simulink model "final_robot_model"  (R2023b)
settings: Solver=VariableStepAuto  StartTime=0.0  StopTime=10.0  RelTol=1e-3
values from neighbouring files (symbols this model uses):
  acceleration_limit = 3    [parameters.m]
  D = 0.93e-6    (= 9.3e-07)    [parameters.m]
  dist0 = 0    [parameters.m]
  gear = 9.6    [parameters.m]
  heading_ref = 0.9    [parameters.m]    (also in set_and_go.m = deg2rad(heading_ref_deg))
  J = 1.01e-6    (= 1.01e-06)    [parameters.m]
  Kb = 0.0074    [parameters.m]
  Kt = Kb    (= 0.0074)    [parameters.m]
  L = 4.1e-3    (= 0.0041)    [parameters.m]
  M = 0.95    [parameters.m]
  path = path .* 0.1    [parameters.m]
  R = 4.1    [parameters.m]
  theta0 = 0    [parameters.m]
  transport_delay = 0.01    [parameters.m]
  Ts = 0.004    [parameters.m]
  turn_acc_limit = 5    [parameters.m]
  vel_ref = 0.5    [parameters.m]
  wheel_distance = 0.147    [parameters.m]
  wrad = 0.03    [parameters.m]
  wzi = (0.065)^2 * M    (= 0.00401375)    [parameters.m]
  x0 = 0    [parameters.m]    (also in plot_trajectory.m = evalin("base", "x0"))
  y0 = 0    [parameters.m]    (also in plot_trajectory.m = evalin("base", "y0"))
undefined symbols (not defined in the file or in its folder): alpha, alpha_heading, Ki, Ki_heading, Ki_turnrate, Kp, Kp_heading, Kp_turnrate, taud, taud_heading
settings Model: Creator=Gianluca  LastModifiedBy=simone

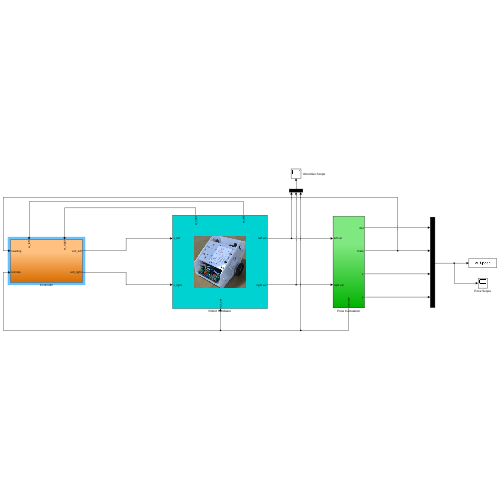
[thumbnail: Simulink's stored preview of the top-level diagram]
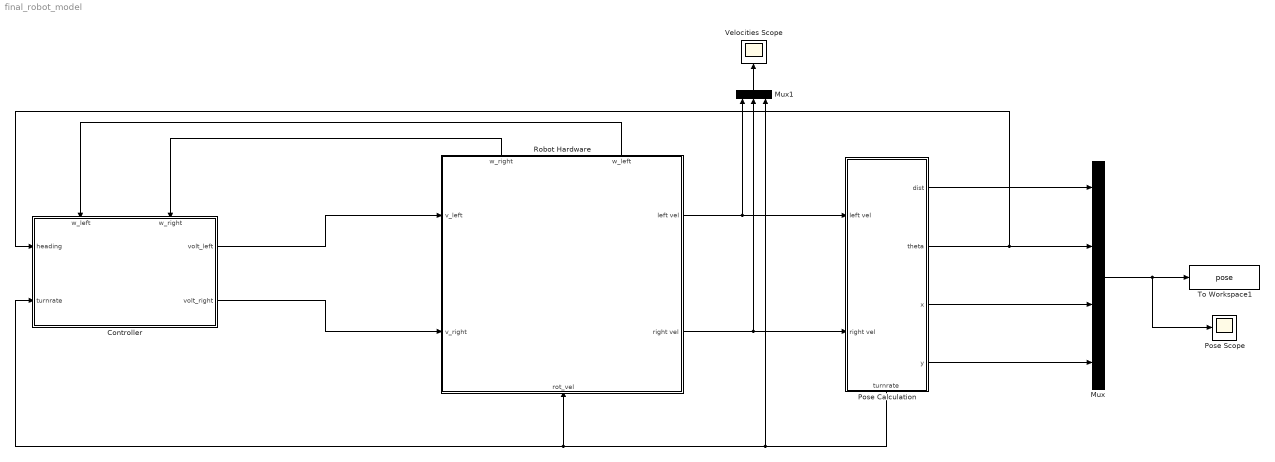
== system final_robot_model ==
  Controller : Subsystem
      settings: PortSchema="{\"entries\":[{\"content\":{\"sides\":[{\"content\":{\"connectorIds\":[\"In1\",\"In2\"]},\"type\":\"ConnectorPlacement.EquallySpacedRectSide\",\"uuid\":\"3d11a138-6336-4e96-9bd3-dfa953b9eab0\"},{\"content\":{\"connectorIds\":[\"Out1\",\"Out2\"],\"side\":\"RIGHT\"},\"type\":\"ConnectorPlacement.EquallySpacedRectSide\",\"uuid\":\"de9a8172-5842-4792-a376-2910158aed35\"},{\"content\":{\"connectorIds\":[\"In3\",\"In4\"],\"side\":\"TOP\"},\"type\":\"ConnectorPlacement.EquallySpacedRectSide\",\"uuid\":\"81659c89-c220-4746-8992-e8ba86bf75e6\"},{\"content\":{\"side\":\"BOTTOM\"},\"type\":\"ConnectorPlacement.EquallySpacedRectSide\",\"uuid\":\"e4167768-df9a-443c-9e0f-b27adaafe9f8\"}]},\"type\":\"ConnectorPlacement.EquallySpacedConnector\",\"uuid\":\"b42d2ec0-7f18-44e6-b925-f5795e7bb3dd\"}],\"packageUris\":[\"http://schema.mathworks.com/mf0/Connector/R2020b\"],\"version\":\"1.0\"}"
  Mux : Mux
  Mux1 : Mux  Inputs=3
  Pose Calculation : Subsystem
      settings: PortSchema="{\"entries\":[{\"content\":{\"sides\":[{\"content\":{\"connectorIds\":[\"In1\",\"In2\"]},\"type\":\"ConnectorPlacement.EquallySpacedRectSide\",\"uuid\":\"46289eb4-3bbb-404a-99f0-e253fad6e87f\"},{\"content\":{\"connectorIds\":[\"Out1\",\"Out2\",\"Out3\",\"Out4\"],\"side\":\"RIGHT\"},\"type\":\"ConnectorPlacement.EquallySpacedRectSide\",\"uuid\":\"ccfc4e76-4e0e-4fcd-8da4-ce03e19c701c\"},{\"content\":{\"side\":\"TOP\"},\"type\":\"ConnectorPlacement.EquallySpacedRectSide\",\"uuid\":\"be5e5684-5a07-4d94-a4cd-7af4c2fd824b\"},{\"content\":{\"connectorIds\":[\"Out5\"],\"side\":\"BOTTOM\"},\"type\":\"ConnectorPlacement.EquallySpacedRectSide\",\"uuid\":\"f3a7bad1-4db8-4eb0-a537-6e6993dfbfe6\"}]},\"type\":\"ConnectorPlacement.EquallySpacedConnector\",\"uuid\":\"6a4a9bee-79c3-4932-b89c-a6fb8d0f2d92\"}],\"packageUris\":[\"http://schema.mathworks.com/mf0/Connector/R2020b\"],\"version\":\"1.0\"}"
  Pose Scope : Scope
  Robot Hardware : Subsystem
      settings: PortSchema="{\"entries\":[{\"content\":{\"sides\":[{\"content\":{\"connectorIds\":[\"In1\",\"In2\"]},\"type\":\"ConnectorPlacement.EquallySpacedRectSide\",\"uuid\":\"419fea77-f9ca-4e06-bea6-681a18650ab8\"},{\"content\":{\"connectorIds\":[\"Out1\",\"Out2\"],\"side\":\"RIGHT\"},\"type\":\"ConnectorPlacement.EquallySpacedRectSide\",\"uuid\":\"1629cad4-6101-470f-acc1-fad0cb327def\"},{\"content\":{\"connectorIds\":[\"Out3\",\"Out4\"],\"side\":\"TOP\"},\"type\":\"ConnectorPlacement.EquallySpacedRectSide\",\"uuid\":\"70c90e71-c188-4b9c-b220-781da08827f9\"},{\"content\":{\"connectorIds\":[\"In3\"],\"side\":\"BOTTOM\"},\"type\":\"ConnectorPlacement.EquallySpacedRectSide\",\"uuid\":\"6ff6b814-ff30-4b88-82ef-7ebf956f2560\"}]},\"type\":\"ConnectorPlacement.EquallySpacedConnector\",\"uuid\":\"ad56978f-143c-418e-863d-6c6f1f6f5d0c\"}],\"packageUris\":[\"http://schema.mathworks.com/mf0/Connector/R2020b\"],\"version\":\"1.0\"}"
      mask Display: image('regbot.png');
  To Workspace1 : ToWorkspace  VariableName=pose  SaveFormat=Timeseries  SampleTime=-1
  Velocities Scope : Scope
  wires:
  Pose Calculation/5(turnrate) -> Mux1/3, Robot Hardware/3(rot_vel), Controller/2(turnrate)
  Mux/1 -> To Workspace1/1, Pose Scope/1
  Pose Calculation/2(theta) -> Mux/2, Controller/1(heading)
  Pose Calculation/1(dist) -> Mux/1
  Mux1/1 -> Velocities Scope/1
  Pose Calculation/3(x) -> Mux/3
  Pose Calculation/4(y) -> Mux/4
  Robot Hardware/4(w_left) -> Controller/3(w_left)
  Robot Hardware/3(w_right) -> Controller/4(w_right)
  Controller/1(volt_left) -> Robot Hardware/1(v_left)
  Controller/2(volt_right) -> Robot Hardware/2(v_right)
  Robot Hardware/1(left vel) -> Pose Calculation/1(left vel), Mux1/1
  Robot Hardware/2(right vel) -> Pose Calculation/2(right vel), Mux1/2

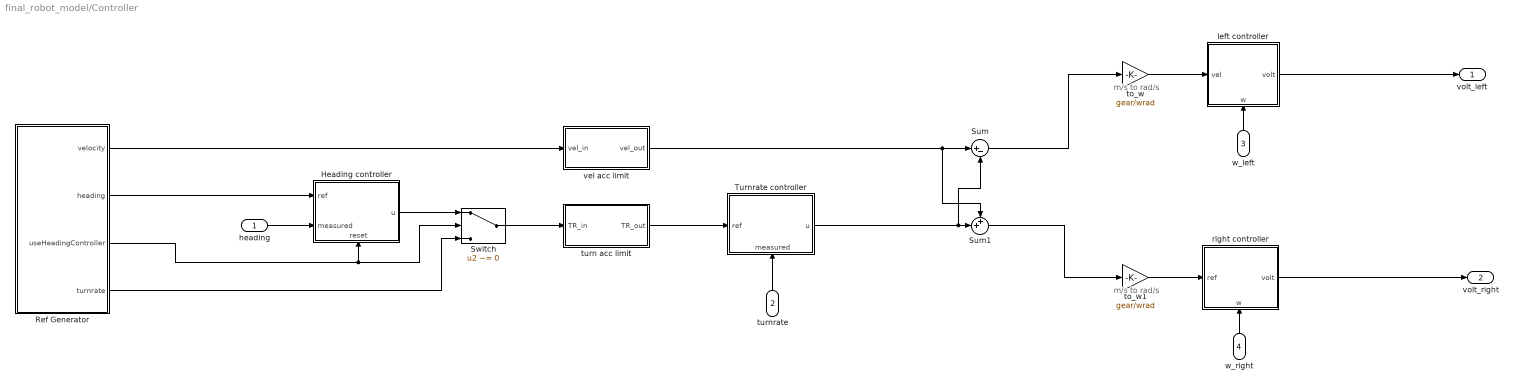
== system final_robot_model/Controller ==
  note: m/s to rad/s
  note: m/s to rad/s
  heading : Inport
  turnrate : Inport  Port=2
  w_left : Inport  Port=3
  w_right : Inport  Port=4
  Heading controller : Subsystem
      settings: PortSchema="{\"entries\":[{\"content\":{\"sides\":[{\"content\":{\"connectorIds\":[\"In1\",\"In2\"]},\"type\":\"ConnectorPlacement.EquallySpacedRectSide\",\"uuid\":\"3bde791d-a2ac-4d13-a51a-30874ee8f75a\"},{\"content\":{\"connectorIds\":[\"Out1\"],\"side\":\"RIGHT\"},\"type\":\"ConnectorPlacement.EquallySpacedRectSide\",\"uuid\":\"88ae4683-d3e7-483e-be55-3d26372f5fe2\"},{\"content\":{\"side\":\"TOP\"},\"type\":\"ConnectorPlacement.EquallySpacedRectSide\",\"uuid\":\"26752a72-f697-4de9-9dcd-1ca4cee0df39\"},{\"content\":{\"connectorIds\":[\"In3\"],\"side\":\"BOTTOM\"},\"type\":\"ConnectorPlacement.EquallySpacedRectSide\",\"uuid\":\"98a7b674-7c45-4a73-92a3-8750bdde1f36\"}]},\"type\":\"ConnectorPlacement.EquallySpacedConnector\",\"uuid\":\"d259c3e3-c5d7-42b6-881b-3a633aa969c6\"}],\"packageUris\":[\"http://schema.mathworks.com/mf0/Connector/R2020b\"],\"version\":\"1.0\"}"
  Ref Generator : Subsystem
  Sum : Sum  Inputs=|+-
  Sum1 : Sum  Inputs=++|
  Switch : Switch  Criteria=u2 ~= 0  Threshold=-999999  SaturateOnIntegerOverflow=off  InputSameDT=off
  Turnrate controller : Subsystem
      settings: PortSchema="{\"entries\":[{\"content\":{\"sides\":[{\"content\":{\"connectorIds\":[\"In1\"]},\"type\":\"ConnectorPlacement.EquallySpacedRectSide\",\"uuid\":\"3bde791d-a2ac-4d13-a51a-30874ee8f75a\"},{\"content\":{\"connectorIds\":[\"Out1\"],\"side\":\"RIGHT\"},\"type\":\"ConnectorPlacement.EquallySpacedRectSide\",\"uuid\":\"88ae4683-d3e7-483e-be55-3d26372f5fe2\"},{\"content\":{\"side\":\"TOP\"},\"type\":\"ConnectorPlacement.EquallySpacedRectSide\",\"uuid\":\"26752a72-f697-4de9-9dcd-1ca4cee0df39\"},{\"content\":{\"connectorIds\":[\"In2\"],\"side\":\"BOTTOM\"},\"type\":\"ConnectorPlacement.EquallySpacedRectSide\",\"uuid\":\"98a7b674-7c45-4a73-92a3-8750bdde1f36\"}]},\"type\":\"ConnectorPlacement.EquallySpacedConnector\",\"uuid\":\"d259c3e3-c5d7-42b6-881b-3a633aa969c6\"}],\"packageUris\":[\"http://schema.mathworks.com/mf0/Connector/R2020b\"],\"version\":\"1.0\"}"
  left controller : Subsystem
      settings: PortSchema="{\"entries\":[{\"content\":{\"sides\":[{\"content\":{\"connectorIds\":[\"In1\"]},\"type\":\"ConnectorPlacement.EquallySpacedRectSide\",\"uuid\":\"3bde791d-a2ac-4d13-a51a-30874ee8f75a\"},{\"content\":{\"connectorIds\":[\"Out1\"],\"side\":\"RIGHT\"},\"type\":\"ConnectorPlacement.EquallySpacedRectSide\",\"uuid\":\"88ae4683-d3e7-483e-be55-3d26372f5fe2\"},{\"content\":{\"side\":\"TOP\"},\"type\":\"ConnectorPlacement.EquallySpacedRectSide\",\"uuid\":\"26752a72-f697-4de9-9dcd-1ca4cee0df39\"},{\"content\":{\"connectorIds\":[\"In2\"],\"side\":\"BOTTOM\"},\"type\":\"ConnectorPlacement.EquallySpacedRectSide\",\"uuid\":\"8837b86a-35cd-4679-9975-e69b760c287c\"}]},\"type\":\"ConnectorPlacement.EquallySpacedConnector\",\"uuid\":\"d259c3e3-c5d7-42b6-881b-3a633aa969c6\"}],\"packageUris\":[\"http://schema.mathworks.com/mf0/Connector/R2020b\"],\"version\":\"1.0\"}"
  right controller : Subsystem
      settings: PortSchema="{\"entries\":[{\"content\":{\"sides\":[{\"content\":{\"connectorIds\":[\"In1\"]},\"type\":\"ConnectorPlacement.EquallySpacedRectSide\",\"uuid\":\"3bde791d-a2ac-4d13-a51a-30874ee8f75a\"},{\"content\":{\"connectorIds\":[\"Out1\"],\"side\":\"RIGHT\"},\"type\":\"ConnectorPlacement.EquallySpacedRectSide\",\"uuid\":\"88ae4683-d3e7-483e-be55-3d26372f5fe2\"},{\"content\":{\"side\":\"TOP\"},\"type\":\"ConnectorPlacement.EquallySpacedRectSide\",\"uuid\":\"26752a72-f697-4de9-9dcd-1ca4cee0df39\"},{\"content\":{\"connectorIds\":[\"In2\"],\"side\":\"BOTTOM\"},\"type\":\"ConnectorPlacement.EquallySpacedRectSide\",\"uuid\":\"1adabdfb-f360-4bb8-8b57-8160c74899b3\"}]},\"type\":\"ConnectorPlacement.EquallySpacedConnector\",\"uuid\":\"d259c3e3-c5d7-42b6-881b-3a633aa969c6\"}],\"packageUris\":[\"http://schema.mathworks.com/mf0/Connector/R2020b\"],\"version\":\"1.0\"}"
  to_w : Gain  Gain=gear/wrad
  to_w1 : Gain  Gain=gear/wrad
  turn acc limit : Subsystem
  vel acc limit : Subsystem
  volt_left : Outport
  volt_right : Outport  Port=2
  wires:
  turn acc limit/1(TR_out) -> Turnrate controller/1(ref)
  left controller/1(volt) -> volt_left/1
  Turnrate controller/1(u) -> Sum/2, Sum1/2
  heading/1 -> Heading controller/2(measured)
  to_w/1 -> left controller/1(vel)
  Sum/1 -> to_w/1
  w_right/1 -> right controller/2(w)
  turnrate/1 -> Turnrate controller/2(measured)
  to_w1/1 -> right controller/1(ref)
  right controller/1(volt) -> volt_right/1
  Sum1/1 -> to_w1/1
  w_left/1 -> left controller/2(w)
  vel acc limit/1(vel_out) -> Sum1/1, Sum/1
  Ref Generator/2(heading) -> Heading controller/1(ref)
  Heading controller/1(u) -> Switch/1
  Switch/1 -> turn acc limit/1(TR_in)
  Ref Generator/4(turnrate) -> Switch/3
  Ref Generator/3(useHeadingController) -> Switch/2, Heading controller/3(reset)
  Ref Generator/1(velocity) -> vel acc limit/1(vel_in)

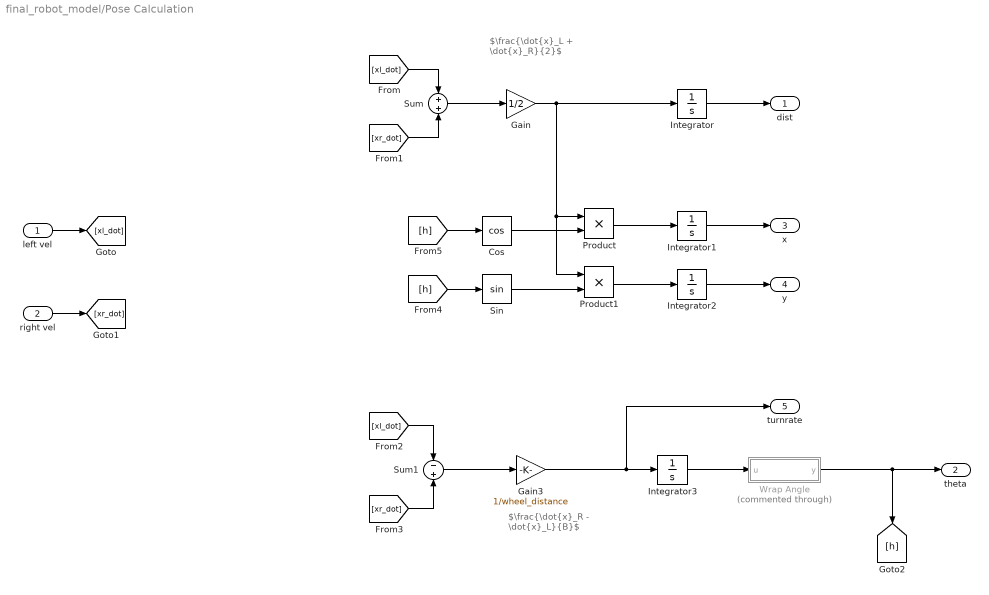
== system final_robot_model/Pose Calculation ==
  note: $\frac{\dot{x}_L + \dot{x}_R}{2}$
  note: $\frac{\dot{x}_R - \dot{x}_L}{B}$
  left vel : Inport
  right vel : Inport  Port=2
  Cos : Trigonometry  Operator=cos
  Gain : Gain  Gain=1/2
  Gain3 : Gain  Gain=1/wheel_distance
  Integrator : Integrator  InitialCondition=dist0
  Integrator1 : Integrator  InitialCondition=x0
  Integrator2 : Integrator  InitialCondition=y0
  Integrator3 : Integrator  InitialCondition=theta0
  Product : Product
  Product1 : Product
  Sin : Trigonometry
  Sum : Sum  Inputs=+|+
  Sum1 : Sum  Inputs=-|+
  Wrap Angle : MATLAB Function  Commented=through  TreatAsAtomicUnit=on
  dist : Outport
  theta : Outport  Port=2
  x : Outport  Port=3
  y : Outport  Port=4
  turnrate : Outport  Port=5
  wires:
  Sum/1 -> Gain/1
  Gain/1 -> Integrator/1, Product/1, Product1/1
  Integrator/1 -> dist/1
  left vel/1 -> [xl_dot]
  right vel/1 -> [xr_dot]
  [xl_dot] -> Sum/1
  [xr_dot] -> Sum/2
  [xl_dot] -> Sum1/1
  [xr_dot] -> Sum1/2
  Gain3/1 -> turnrate/1, Integrator3/1
  Sum1/1 -> Gain3/1
  [h] -> Sin/1
  Integrator2/1 -> y/1
  Integrator1/1 -> x/1
  [h] -> Cos/1
  Sin/1 -> Product1/2
  Cos/1 -> Product/2
  Product1/1 -> Integrator2/1
  Product/1 -> Integrator1/1
  Integrator3/1 -> Wrap Angle/1(u)
  Wrap Angle/1(y) -> [h], theta/1

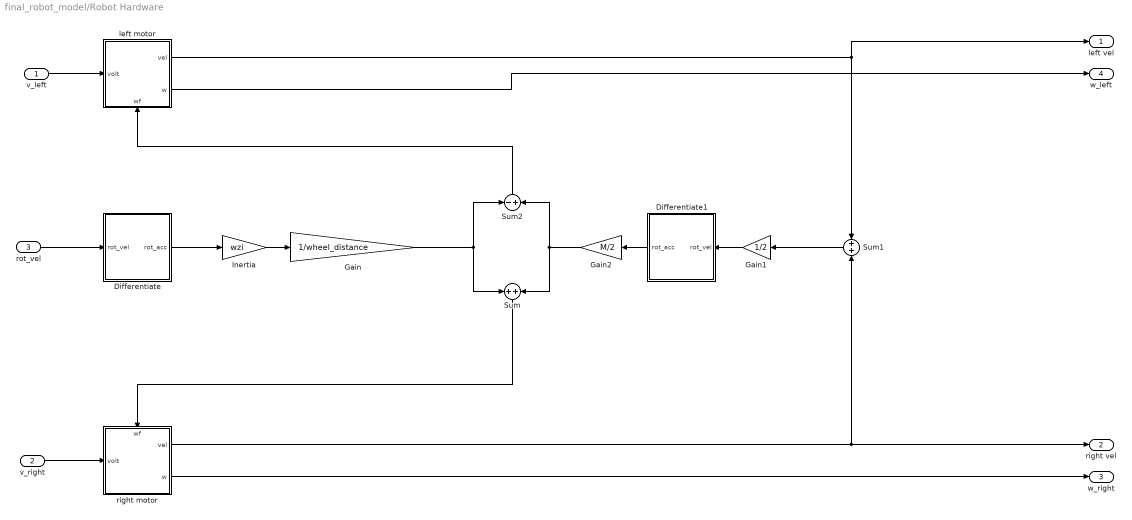
== system final_robot_model/Robot Hardware ==
  v_left : Inport
  v_right : Inport  Port=2
  rot_vel : Inport  Port=3
  Differentiate : Subsystem
  Differentiate1 : Subsystem
  Gain : Gain  Gain=1/wheel_distance
  Gain1 : Gain  Gain=1/2
  Gain2 : Gain  Gain=M/2
  Inertia : Gain  Gain=wzi
  Sum : Sum  Inputs=+|+
  Sum1 : Sum  Inputs=+|+
  Sum2 : Sum  Inputs=-|+
  left motor : Subsystem
      settings: PortSchema="{\"entries\":[{\"content\":{\"sides\":[{\"content\":{\"connectorIds\":[\"In1\"]},\"type\":\"ConnectorPlacement.EquallySpacedRectSide\",\"uuid\":\"3bde791d-a2ac-4d13-a51a-30874ee8f75a\"},{\"content\":{\"connectorIds\":[\"Out1\",\"Out2\"],\"side\":\"RIGHT\"},\"type\":\"ConnectorPlacement.EquallySpacedRectSide\",\"uuid\":\"88ae4683-d3e7-483e-be55-3d26372f5fe2\"},{\"content\":{\"side\":\"TOP\"},\"type\":\"ConnectorPlacement.EquallySpacedRectSide\",\"uuid\":\"26752a72-f697-4de9-9dcd-1ca4cee0df39\"},{\"content\":{\"connectorIds\":[\"In2\"],\"side\":\"BOTTOM\"},\"type\":\"ConnectorPlacement.EquallySpacedRectSide\",\"uuid\":\"bdf58d17-97a4-48aa-9393-076eaaeca649\"}]},\"type\":\"ConnectorPlacement.EquallySpacedConnector\",\"uuid\":\"d259c3e3-c5d7-42b6-881b-3a633aa969c6\"}],\"packageUris\":[\"http://schema.mathworks.com/mf0/Connector/R2020b\"],\"version\":\"1.0\"}"
  right motor : Subsystem
      settings: PortSchema="{\"entries\":[{\"content\":{\"sides\":[{\"content\":{\"connectorIds\":[\"In1\"]},\"type\":\"ConnectorPlacement.EquallySpacedRectSide\",\"uuid\":\"3bde791d-a2ac-4d13-a51a-30874ee8f75a\"},{\"content\":{\"connectorIds\":[\"Out1\",\"Out2\"],\"side\":\"RIGHT\"},\"type\":\"ConnectorPlacement.EquallySpacedRectSide\",\"uuid\":\"88ae4683-d3e7-483e-be55-3d26372f5fe2\"},{\"content\":{\"connectorIds\":[\"In2\"],\"side\":\"TOP\"},\"type\":\"ConnectorPlacement.EquallySpacedRectSide\",\"uuid\":\"26752a72-f697-4de9-9dcd-1ca4cee0df39\"},{\"content\":{\"side\":\"BOTTOM\"},\"type\":\"ConnectorPlacement.EquallySpacedRectSide\",\"uuid\":\"bdf58d17-97a4-48aa-9393-076eaaeca649\"}]},\"type\":\"ConnectorPlacement.EquallySpacedConnector\",\"uuid\":\"d259c3e3-c5d7-42b6-881b-3a633aa969c6\"}],\"packageUris\":[\"http://schema.mathworks.com/mf0/Connector/R2020b\"],\"version\":\"1.0\"}"
  left vel : Outport
  right vel : Outport  Port=2
  w_right : Outport  Port=3
  w_left : Outport  Port=4
  wires:
  v_left/1 -> left motor/1(volt)
  left motor/2(w) -> w_left/1
  v_right/1 -> right motor/1(volt)
  right motor/2(w) -> w_right/1
  rot_vel/1 -> Differentiate/1(rot_vel)
  Differentiate/1(rot_acc) -> Inertia/1
  Inertia/1 -> Gain/1
  Gain/1 -> Sum/1, Sum2/1
  Sum/1 -> right motor/2(wf)
  left motor/1(vel) -> left vel/1, Sum1/1
  Sum1/1 -> Gain1/1
  Gain1/1 -> Differentiate1/1(rot_vel)
  Differentiate1/1(rot_acc) -> Gain2/1
  Sum2/1 -> left motor/2(wf)
  right motor/1(vel) -> right vel/1, Sum1/2
  Gain2/1 -> Sum2/2, Sum/2

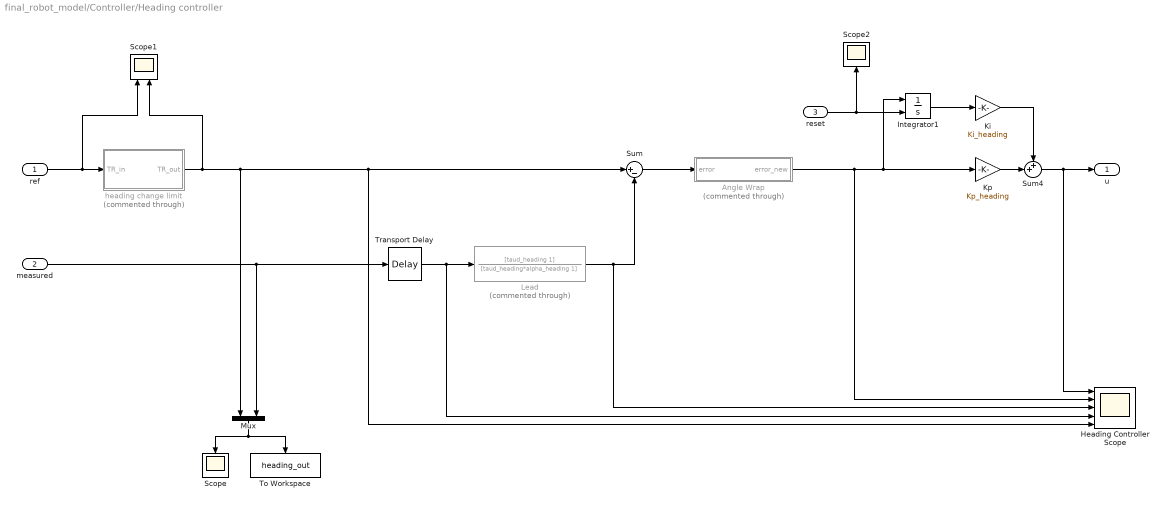
== system final_robot_model/Controller/Heading controller ==
  ref : Inport
  measured : Inport  Port=2
  reset : Inport  Port=3
  Angle Wrap : MATLAB Function  Commented=through  TreatAsAtomicUnit=on
  Heading Controller Scope : Scope  NumInputPorts=5
  Integrator1 : Integrator  ExternalReset=either
  Ki : Gain  Gain=Ki_heading
  Kp : Gain  Gain=Kp_heading
  Lead : TransferFcn  Commented=through  Numerator=[taud_heading 1]  Denominator=[taud_heading*alpha_heading 1]
  Mux : Mux  Inputs=2
  Scope : Scope
  Scope1 : Scope  NumInputPorts=2
  Scope2 : Scope
  Sum : Sum  Inputs=|+-
  Sum4 : Sum  Inputs=++|
  To Workspace : ToWorkspace  VariableName=heading_out  SaveFormat=Timeseries  SampleTime=-1
  Transport Delay : TransportDelay  DelayTime=transport_delay
  heading change limit : Subsystem  Commented=through
  u : Outport
  wires:
  ref/1 -> Scope1/1, heading change limit/1(TR_in)
  measured/1 -> Transport Delay/1, Mux/2
  Transport Delay/1 -> Heading Controller Scope/4, Lead/1
  Sum4/1 -> Heading Controller Scope/1, u/1
  Sum/1 -> Angle Wrap/1(error)
  Integrator1/1 -> Ki/1
  Ki/1 -> Sum4/1
  Kp/1 -> Sum4/2
  Mux/1 -> To Workspace/1, Scope/1
  Lead/1 -> Sum/2, Heading Controller Scope/3
  heading change limit/1(TR_out) -> Heading Controller Scope/5, Sum/1, Mux/1, Scope1/2
  reset/1 -> Integrator1/2, Scope2/1
  Angle Wrap/1(error_new) -> Heading Controller Scope/2, Integrator1/1, Kp/1

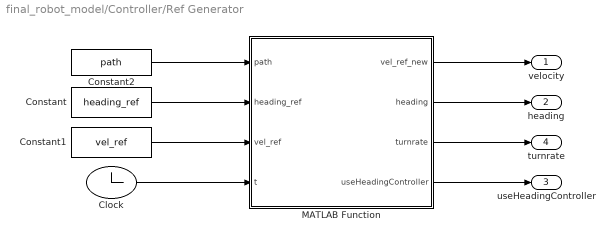
== system final_robot_model/Controller/Ref Generator ==
  Clock : Clock
  Constant : Constant  Value=heading_ref
  Constant1 : Constant  Value=vel_ref
  Constant2 : Constant  Value=path
  MATLAB Function : MATLAB Function  TreatAsAtomicUnit=on
  velocity : Outport
  heading : Outport  Port=2
  useHeadingController : Outport  Port=3
  turnrate : Outport  Port=4
  wires:
  Clock/1 -> MATLAB Function/4(t)
  Constant/1 -> MATLAB Function/2(heading_ref)
  Constant1/1 -> MATLAB Function/3(vel_ref)
  MATLAB Function/2(heading) -> heading/1
  Constant2/1 -> MATLAB Function/1(path)
  MATLAB Function/3(turnrate) -> turnrate/1
  MATLAB Function/4(useHeadingController) -> useHeadingController/1
  MATLAB Function/1(vel_ref_new) -> velocity/1

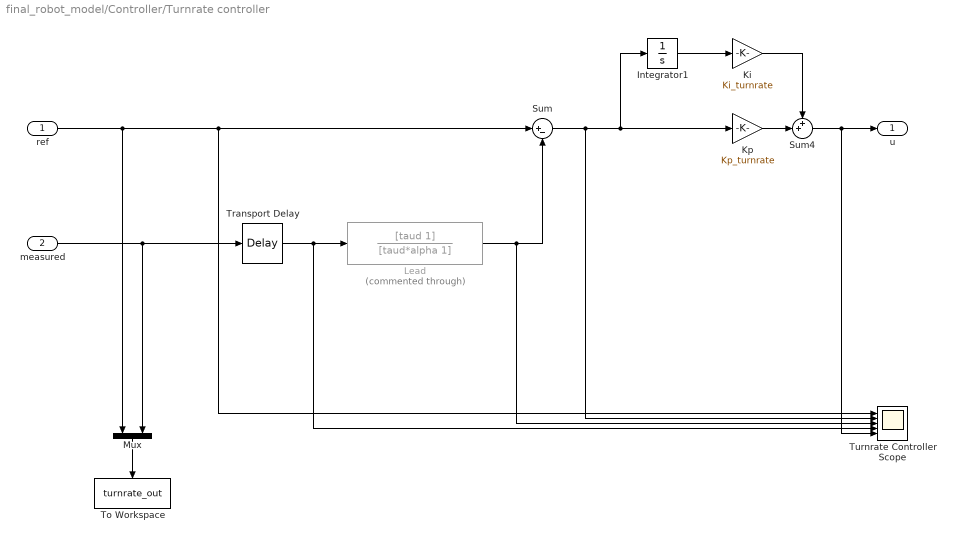
== system final_robot_model/Controller/Turnrate controller ==
  ref : Inport
  measured : Inport  Port=2
  Integrator1 : Integrator
  Ki : Gain  Gain=Ki_turnrate
  Kp : Gain  Gain=Kp_turnrate
  Lead : TransferFcn  Commented=through  Numerator=[taud 1]  Denominator=[taud*alpha 1]
  Mux : Mux  Inputs=2
  Sum : Sum  Inputs=|+-
  Sum4 : Sum  Inputs=++|
  To Workspace : ToWorkspace  VariableName=turnrate_out  SaveFormat=Timeseries  SampleTime=-1
  Transport Delay : TransportDelay  DelayTime=transport_delay
  Turnrate Controller Scope : Scope  NumInputPorts=5
  u : Outport
  wires:
  ref/1 -> Turnrate Controller Scope/1, Sum/1, Mux/1
  Lead/1 -> Sum/2, Turnrate Controller Scope/3
  measured/1 -> Transport Delay/1, Mux/2
  Transport Delay/1 -> Turnrate Controller Scope/4, Lead/1
  Sum4/1 -> Turnrate Controller Scope/5, u/1
  Sum/1 -> Turnrate Controller Scope/2, Integrator1/1, Kp/1
  Integrator1/1 -> Ki/1
  Ki/1 -> Sum4/1
  Kp/1 -> Sum4/2
  Mux/1 -> To Workspace/1

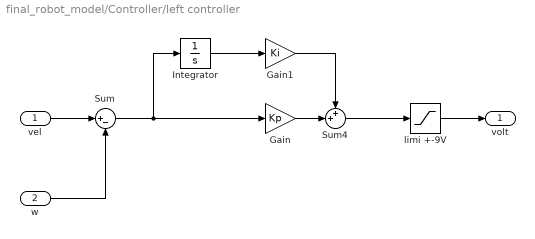
== system final_robot_model/Controller/left controller ==
  vel : Inport
  w : Inport  Port=2
  Gain : Gain  Gain=Kp
  Gain1 : Gain  Gain=Ki
  Integrator : Integrator
  Sum : Sum  Inputs=|+-
  Sum4 : Sum  Inputs=++|
  limi +-9V : Saturate  UpperLimit=9  LowerLimit=-9
  volt : Outport
  wires:
  Gain/1 -> Sum4/2
  Integrator/1 -> Gain1/1
  Gain1/1 -> Sum4/1
  vel/1 -> Sum/1
  w/1 -> Sum/2
  Sum/1 -> Integrator/1, Gain/1
  Sum4/1 -> limi +-9V/1
  limi +-9V/1 -> volt/1

== system final_robot_model/Controller/right controller ==
  ref : Inport
  w : Inport  Port=2
  Gain2 : Gain  Gain=Kp
  Gain3 : Gain  Gain=Ki
  Integrator1 : Integrator
  Sum : Sum  Inputs=|+-
  Sum1 : Sum  Inputs=++|
  limi +-9V : Saturate  UpperLimit=9  LowerLimit=-9
  volt : Outport
  wires:
  Integrator1/1 -> Gain3/1
  Gain2/1 -> Sum1/2
  Gain3/1 -> Sum1/1
  Sum/1 -> Integrator1/1, Gain2/1
  ref/1 -> Sum/1
  w/1 -> Sum/2
  Sum1/1 -> limi +-9V/1
  limi +-9V/1 -> volt/1

== system final_robot_model/Controller/turn acc limit ==
  TR_in : Inport
  Gain : Gain  Gain=100
  Integrator : Integrator
  Saturation : Saturate  UpperLimit=turn_acc_limit  LowerLimit=-turn_acc_limit
  Sum : Sum  Inputs=|+-
  TR_out : Outport
  wires:
  TR_in/1 -> Sum/1
  Sum/1 -> Gain/1
  Gain/1 -> Saturation/1
  Saturation/1 -> Integrator/1
  Integrator/1 -> Sum/2, TR_out/1

== system final_robot_model/Controller/vel acc limit ==
  vel_in : Inport
  Gain : Gain  Gain=100
  Integrator : Integrator
  Saturation : Saturate  UpperLimit=acceleration_limit  LowerLimit=-acceleration_limit
  Sum : Sum  Inputs=|+-
  vel_out : Outport
  wires:
  vel_in/1 -> Sum/1
  Sum/1 -> Gain/1
  Gain/1 -> Saturation/1
  Saturation/1 -> Integrator/1
  Integrator/1 -> Sum/2, vel_out/1

== system final_robot_model/Robot Hardware/Differentiate ==
  rot_vel : Inport
  Gain : Gain  Gain=100
  Integrator : Integrator
  Sum : Sum  Inputs=|+-
  rot_acc : Outport
  wires:
  rot_vel/1 -> Sum/1
  Sum/1 -> Gain/1
  Integrator/1 -> Sum/2
  Gain/1 -> rot_acc/1, Integrator/1

== system final_robot_model/Robot Hardware/Differentiate1 ==
  rot_vel : Inport
  Gain : Gain  Gain=100
  Integrator : Integrator
  Sum : Sum  Inputs=|+-
  rot_acc : Outport
  wires:
  rot_vel/1 -> Sum/1
  Sum/1 -> Gain/1
  Integrator/1 -> Sum/2
  Gain/1 -> rot_acc/1, Integrator/1

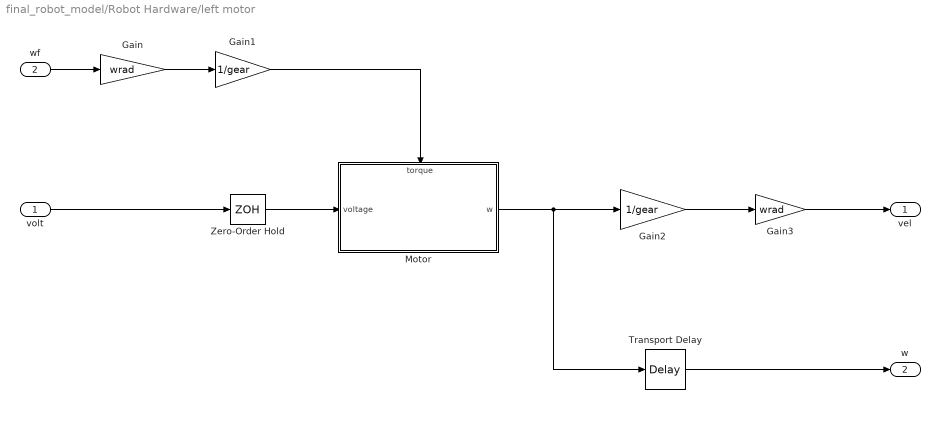
== system final_robot_model/Robot Hardware/left motor ==
  volt : Inport
  wf : Inport  Port=2
  Gain : Gain  Gain=wrad
  Gain1 : Gain  Gain=1/gear
  Gain2 : Gain  Gain=1/gear
  Gain3 : Gain  Gain=wrad
  Motor : Subsystem
      settings: PortSchema="{\"entries\":[{\"content\":{\"sides\":[{\"content\":{\"connectorIds\":[\"In1\"]},\"type\":\"ConnectorPlacement.EquallySpacedRectSide\",\"uuid\":\"3bde791d-a2ac-4d13-a51a-30874ee8f75a\"},{\"content\":{\"connectorIds\":[\"Out1\"],\"side\":\"RIGHT\"},\"type\":\"ConnectorPlacement.EquallySpacedRectSide\",\"uuid\":\"88ae4683-d3e7-483e-be55-3d26372f5fe2\"},{\"content\":{\"connectorIds\":[\"In2\"],\"side\":\"TOP\"},\"type\":\"ConnectorPlacement.EquallySpacedRectSide\",\"uuid\":\"26752a72-f697-4de9-9dcd-1ca4cee0df39\"}]},\"type\":\"ConnectorPlacement.EquallySpacedConnector\",\"uuid\":\"d259c3e3-c5d7-42b6-881b-3a633aa969c6\"}],\"packageUris\":[\"http://schema.mathworks.com/mf0/Connector/R2020b\"],\"version\":\"1.0\"}"
  Transport Delay : TransportDelay  DelayTime=transport_delay
  Zero-Order Hold : ZeroOrderHold  SampleTime=Ts
  vel : Outport
  w : Outport  Port=2
  wires:
  wf/1 -> Gain/1
  Gain/1 -> Gain1/1
  Gain1/1 -> Motor/2(torque)
  Gain3/1 -> vel/1
  Gain2/1 -> Gain3/1
  Motor/1(w) -> Transport Delay/1, Gain2/1
  Transport Delay/1 -> w/1
  volt/1 -> Zero-Order Hold/1
  Zero-Order Hold/1 -> Motor/1(voltage)

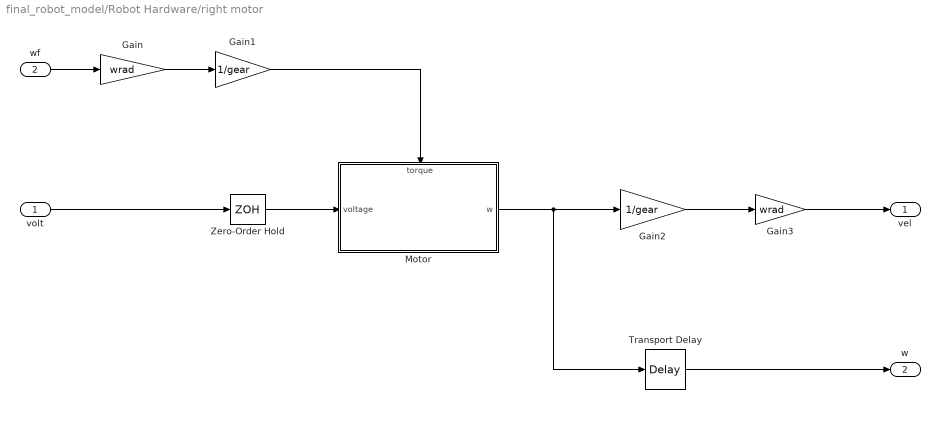
== system final_robot_model/Robot Hardware/right motor ==
  volt : Inport
  wf : Inport  Port=2
  Gain : Gain  Gain=wrad
  Gain1 : Gain  Gain=1/gear
  Gain2 : Gain  Gain=1/gear
  Gain3 : Gain  Gain=wrad
  Motor : Subsystem
      settings: PortSchema="{\"entries\":[{\"content\":{\"sides\":[{\"content\":{\"connectorIds\":[\"In1\"]},\"type\":\"ConnectorPlacement.EquallySpacedRectSide\",\"uuid\":\"3bde791d-a2ac-4d13-a51a-30874ee8f75a\"},{\"content\":{\"connectorIds\":[\"Out1\"],\"side\":\"RIGHT\"},\"type\":\"ConnectorPlacement.EquallySpacedRectSide\",\"uuid\":\"88ae4683-d3e7-483e-be55-3d26372f5fe2\"},{\"content\":{\"connectorIds\":[\"In2\"],\"side\":\"TOP\"},\"type\":\"ConnectorPlacement.EquallySpacedRectSide\",\"uuid\":\"26752a72-f697-4de9-9dcd-1ca4cee0df39\"}]},\"type\":\"ConnectorPlacement.EquallySpacedConnector\",\"uuid\":\"d259c3e3-c5d7-42b6-881b-3a633aa969c6\"}],\"packageUris\":[\"http://schema.mathworks.com/mf0/Connector/R2020b\"],\"version\":\"1.0\"}"
  Transport Delay : TransportDelay  DelayTime=transport_delay
  Zero-Order Hold : ZeroOrderHold  SampleTime=Ts
  vel : Outport
  w : Outport  Port=2
  wires:
  wf/1 -> Gain/1
  Gain/1 -> Gain1/1
  Gain1/1 -> Motor/2(torque)
  Gain3/1 -> vel/1
  Gain2/1 -> Gain3/1
  Motor/1(w) -> Transport Delay/1, Gain2/1
  Transport Delay/1 -> w/1
  volt/1 -> Zero-Order Hold/1
  Zero-Order Hold/1 -> Motor/1(voltage)

== system final_robot_model/Controller/Heading controller/heading change limit ==
  TR_in : Inport
  Gain : Gain  Gain=100
  Integrator : Integrator
  Saturation : Saturate  UpperLimit=turn_acc_limit  LowerLimit=-turn_acc_limit
  Sum : Sum  Inputs=|+-
  TR_out : Outport
  wires:
  TR_in/1 -> Sum/1
  Sum/1 -> Gain/1
  Gain/1 -> Saturation/1
  Saturation/1 -> Integrator/1
  Integrator/1 -> Sum/2, TR_out/1

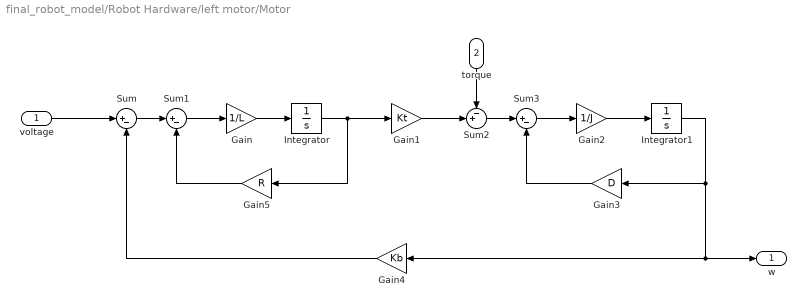
== system final_robot_model/Robot Hardware/left motor/Motor ==
  voltage : Inport
  torque : Inport  Port=2
  Gain : Gain  Gain=1/L
  Gain1 : Gain  Gain=Kt
  Gain2 : Gain  Gain=1/J
  Gain3 : Gain  Gain=D
  Gain4 : Gain  Gain=Kb
  Gain5 : Gain  Gain=R
  Integrator : Integrator
  Integrator1 : Integrator
  Sum : Sum  Inputs=|+-
  Sum1 : Sum  Inputs=|+-
  Sum2 : Sum  Inputs=-+|
  Sum3 : Sum  Inputs=|+-
  w : Outport
  wires:
  voltage/1 -> Sum/1
  Sum/1 -> Sum1/1
  Gain/1 -> Integrator/1
  Gain1/1 -> Sum2/2
  Integrator/1 -> Gain5/1, Gain1/1
  torque/1 -> Sum2/1
  Sum2/1 -> Sum3/1
  Sum3/1 -> Gain2/1
  Gain2/1 -> Integrator1/1
  Integrator1/1 -> Gain3/1, Gain4/1, w/1
  Gain3/1 -> Sum3/2
  Gain4/1 -> Sum/2
  Gain5/1 -> Sum1/2
  Sum1/1 -> Gain/1

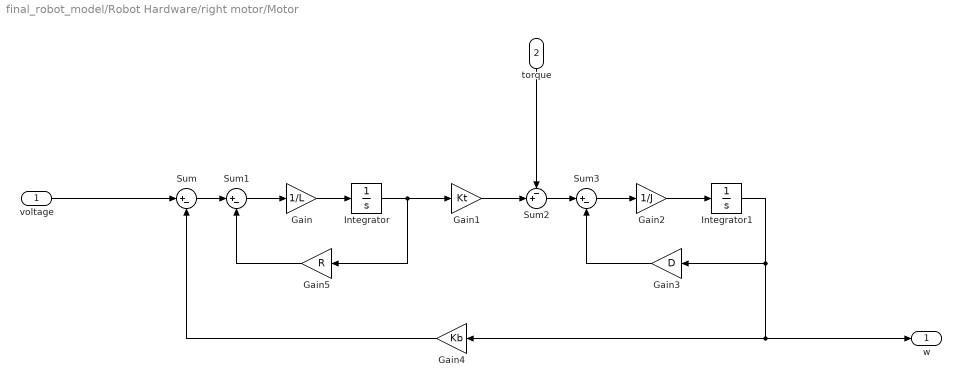
== system final_robot_model/Robot Hardware/right motor/Motor ==
  voltage : Inport
  torque : Inport  Port=2
  Gain : Gain  Gain=1/L
  Gain1 : Gain  Gain=Kt
  Gain2 : Gain  Gain=1/J
  Gain3 : Gain  Gain=D
  Gain4 : Gain  Gain=Kb
  Gain5 : Gain  Gain=R
  Integrator : Integrator
  Integrator1 : Integrator
  Sum : Sum  Inputs=|+-
  Sum1 : Sum  Inputs=|+-
  Sum2 : Sum  Inputs=-+|
  Sum3 : Sum  Inputs=|+-
  w : Outport
  wires:
  voltage/1 -> Sum/1
  Sum/1 -> Sum1/1
  Gain/1 -> Integrator/1
  Gain1/1 -> Sum2/2
  Integrator/1 -> Gain5/1, Gain1/1
  torque/1 -> Sum2/1
  Sum2/1 -> Sum3/1
  Sum3/1 -> Gain2/1
  Gain2/1 -> Integrator1/1
  Integrator1/1 -> Gain3/1, Gain4/1, w/1
  Gain3/1 -> Sum3/2
  Gain4/1 -> Sum/2
  Gain5/1 -> Sum1/2
  Sum1/1 -> Gain/1

== matlab function final_robot_model/Pose Calculation/Wrap Angle ==
  data: u input; y output
function y = wrap_angle(u)

y = wrapToPi(u);

== matlab function final_robot_model/Controller/Ref Generator/MATLAB Function ==
  data: vel_ref_new output; path input; heading_ref input; vel_ref input; heading output size=1; t input; turnrate output; useHeadingController output
function [vel_ref_new, heading, turnrate, useHeadingController] = make_ref(path, heading_ref, vel_ref, t)

% Step
if heading_ref ~= -999999
    vel_ref_new = vel_ref;
    heading = heading_ref;
    turnrate = 0;
    useHeadingController = 1;
% Custom sequence
else
    [vel_ref_new, heading, turnrate, useHeadingController] = get_ref(t, vel_ref, path);
end

end

== matlab function final_robot_model/Controller/Heading controller/Angle Wrap ==
  data: error input; error_new output
function error_new = wrap(error)

if (error < -pi)
    error_new = error + 2*pi;
elseif(error > pi)
    error_new = error - 2*pi;
else
    error_new = error;
end
